simulink library "lic"  (R2021b)
settings: Solver=VariableStepAuto  StartTime=0.0  StopTime=10.0  RelTol=1e-3
undefined symbols (not defined in the file): C_TICK_TIME_S, ENUM_LANEQUALITY_HIGH, ENUM_LANEQUALITY_MEDIUM, ENUM_LFCSTATE_DEGRADED, FALSE, KAPP_VehicleWidth_m, KLIC_C0CrossingThr_m, KLIC_C1Max4Act_rad, KLIC_C2Max4Act_rat, KLIC_C2Max4Disable_rat, KLIC_C2Max4DisableThr_s, KLIC_CalDefaultTLC_s, KLIC_CalTLCMax_s, KLIC_CalTLCMin_s, KLIC_DefaultLaneWidth_m, KLIC_Lane4ActThr_s, KLIC_LaneWidHoldOnTime_s, KLIC_LaneWidRampFinErrThres_m, KLIC_LaneWidRampFinTimeThres_s, KLIC_LaneWidRampInFalRt_mps, KLIC_LaneWidRampInRisRt_mps, KLIC_LaneWidRampOutFalRt_mps, KLIC_LaneWidRampOutRisRt_mps, KLIC_LaneWidthLowThr_m, KLIC_LaneWidthUpThr_m, KLIC_TLCTriggerThrHysis_s, KPER_DefaultLaneWidth_m, MIFO_TLCThr4LKA_s, TRUE
libraries: hcu_lib x33, simulink x8
(part 1 of 2)
settings Model: Creator=power  LastModifiedBy=power

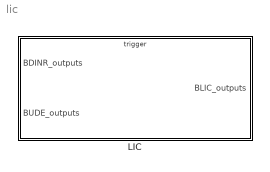
== system lic ==
  LIC : Subsystem

== system lic/LIC ==
  BDINR_outputs : Inport  OutDataTypeStr=Bus: BDINR_outputs
  BUDE_outputs : Inport  Port=2  OutDataTypeStr=Bus: BUDE_outputs
  trig_LIC : TriggerPort  TriggerType=function-call  VariantControl=(inherit)
      settings: AttributesFormatString=State = %<StatesWhenEnabling>
  Bus Creator : BusCreator  Inputs=37  OutDataTypeStr=Bus: BPER_outputs
  Bus Selector1 : BusSelector  OutputSignals=VDINR_CamInternalError_flg,VDINR_LaneQualityL_enum,VDINR_LaneQualityR_enum,VDINR_LaneC0L_m,VDINR_LaneC0R_m,VDINR_LaneC1L_rad,VDINR_LaneC1R_rad,VDINR_LaneC2L_rat,VDINR_LaneC2R_rat,VDINR_LaneC3L_rat,VDINR_LaneC3R_rat,VDINR_TLCL_s,VDINR_TLCLValid_flg,VDINR_TLCR_s,VDINR_TLCRValid_flg,VDINR_VehSpd_mps,VDINR_YawRate_radps,VDINR_ViewRangeEndL_m,VDINR_ViewRangeEndR_m
  Bus Selector2 : BusSelector  OutputSignals=VUDE_NOFTRACKS_num,VUDE_TRACKSX_m,VUDE_TRACKSY_m,VUDE_TRACKSOBST_enum,VUDE_TRACKSVEL_mps,VUDE_TRACKSWIDTH_m,VUDE_TRACKSID_enum,VUDE_TRACKSATT_rad,VUDE_TRACKSEXSPROB_num,VUDE_TRACKSACCEL_mps2,VUDE_RadObjectValid_flg,VUDE_TRACKSRADDYNSTAT_enum,VUDE_CamObstacleValid_flg,VUDE_TRACKSMEDYNSTAT_enum
  lic : Subsystem  TreatAsAtomicUnit=on
  BLIC_outputs : Outport  OutDataTypeStr=Bus: BPER_outputs
  wires:
  Bus Creator/1 -> BLIC_outputs/1  "BLIC_outputs"
  BUDE_outputs/1 -> Bus Selector2/1
  BDINR_outputs/1 -> Bus Selector1/1

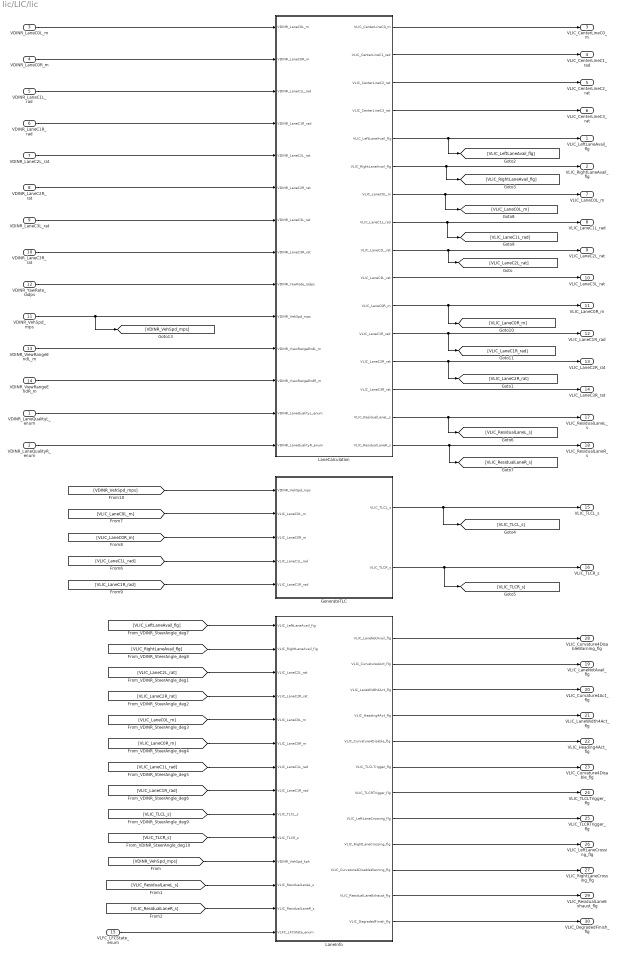
== system lic/LIC/lic ==
  VDINR_LaneQualityL_enum : Inport
  VDINR_LaneQualityR_enum : Inport  Port=2
  VDINR_LaneC0L_m : Inport  Port=3
  VDINR_LaneC0R_m : Inport  Port=4
  VDINR_LaneC1L_rad : Inport  Port=5
  VDINR_LaneC1R_rad : Inport  Port=6
  VDINR_LaneC2L_rat : Inport  Port=7
  VDINR_LaneC2R_rat : Inport  Port=8
  VDINR_LaneC3L_rat : Inport  Port=9
  VDINR_LaneC3R_rat : Inport  Port=10
  VDINR_VehSpd_mps : Inport  Port=11
  VDINR_YawRate_radps : Inport  Port=12
  VDINR_ViewRangeEndL_m : Inport  Port=13
  VDINR_ViewRangeEndR_m : Inport  Port=14
  VLFC_LFCState_enum : Inport  Port=15
  GenerateTLC : Subsystem
  LaneCalculation : Subsystem
  LaneInfo : Subsystem  AncestorBlock=ifo/IFO/ifo/LaneInfo  TreatAsAtomicUnit=on
  VLIC_LeftLaneAvail_flg : Outport
  VLIC_RightLaneAvail_flg : Outport  Port=2
  "VLIC_CenterLineC0_m " : Outport  Port=3
  VLIC_CenterLineC1_rad : Outport  Port=4
  VLIC_CenterLineC2_rat : Outport  Port=5
  VLIC_CenterLineC3_rat : Outport  Port=6
  VLIC_LaneC0L_m : Outport  Port=7
  VLIC_LaneC1L_rad : Outport  Port=8
  VLIC_LaneC2L_rat : Outport  Port=9
  VLIC_LaneC3L_rat : Outport  Port=10
  VLIC_LaneC0R_m : Outport  Port=11
  VLIC_LaneC1R_rad : Outport  Port=12
  VLIC_LaneC2R_rat : Outport  Port=13
  VLIC_LaneC3R_rat : Outport  Port=14
  VLIC_TLCL_s : Outport  Port=15
  VLIC_TLCR_s : Outport  Port=16
  VLIC_ResidualLaneL_s : Outport  Port=17
  VLIC_ResidualLaneR_s : Outport  Port=18
  VLIC_LaneNotAvail_flg : Outport  Port=19
  VLIC_Curvature4Act_flg : Outport  Port=20
  VLIC_LaneWidth4Act_flg : Outport  Port=21
  VLIC_Heading4Act_flg : Outport  Port=22
  VLIC_Curvature4Disable_flg : Outport  Port=23
  VLIC_TLCLTrigger_flg : Outport  Port=24
  VLIC_TLCRTrigger_flg : Outport  Port=25
  VLIC_LeftLaneCrossing_flg : Outport  Port=26
  VLIC_RightLaneCrossing_flg : Outport  Port=27
  VLIC_Curvature4DisableWarning_flg : Outport  Port=28
  VLIC_ResidualLaneExhaust_flg : Outport  Port=29
  VLIC_DegradedFinish_flg : Outport  Port=30
  wires:
  [VDINR_VehSpd_mps] -> GenerateTLC/1(VDINR_VehSpd_mps)
  LaneInfo/1(VLIC_LaneNotAvail_flg) -> VLIC_Curvature4DisableWarning_flg/1
  LaneInfo/10(VLIC_Curvature4DisableWarning_flg) -> VLIC_RightLaneCrossing_flg/1
  LaneInfo/9(VLIC_RightLaneCrossing_flg) -> VLIC_LeftLaneCrossing_flg/1
  LaneInfo/8(VLIC_LeftLaneCrossing_flg) -> VLIC_TLCRTrigger_flg/1
  LaneInfo/7(VLIC_TLCRTrigger_flg) -> VLIC_TLCLTrigger_flg/1
  LaneInfo/6(VLIC_TLCLTrigger_flg) -> VLIC_Curvature4Disable_flg/1
  LaneInfo/5(VLIC_Curvature4Disable_flg) -> VLIC_Heading4Act_flg/1
  LaneInfo/4(VLIC_Heading4Act_flg) -> VLIC_LaneWidth4Act_flg/1
  LaneInfo/3(VLIC_LaneWidth4Act_flg) -> VLIC_Curvature4Act_flg/1
  LaneInfo/2(VLIC_Curvature4Act_flg) -> VLIC_LaneNotAvail_flg/1
  [VDINR_VehSpd_mps] -> LaneInfo/11(VDINR_VehSpd_kph)
  [VLIC_TLCR_s] -> LaneInfo/10(VLIC_TLCR_s)
  [VLIC_TLCL_s] -> LaneInfo/9(VLIC_TLCL_s)
  [VLIC_RightLaneAvail_flg] -> LaneInfo/2("VLIC_RightLaneAvail_fig ")
  [VLIC_LeftLaneAvail_flg] -> LaneInfo/1("VLIC_LeftLaneAvail_fig ")
  [VLIC_LaneC1R_rad] -> LaneInfo/8(VLIC_LaneC1R_rad)
  [VLIC_LaneC1L_rad] -> LaneInfo/7(VLIC_LaneC1L_rad)
  [VLIC_LaneC0R_m] -> LaneInfo/6(VLIC_LaneC0R_m)
  [VLIC_LaneC0L_m] -> LaneInfo/5(VLIC_LaneC0L_m)
  [VLIC_LaneC2R_rat] -> LaneInfo/4(VLIC_LaneC2R_rat)
  [VLIC_LaneC2L_rat] -> LaneInfo/3(VLIC_LaneC2L_rat)
  VDINR_LaneC1L_rad/1 -> LaneCalculation/3(VDINR_LaneC1L_rad)
  VDINR_LaneC2L_rat/1 -> LaneCalculation/5(VDINR_LaneC2L_rat)
  VDINR_LaneC2R_rat/1 -> LaneCalculation/6(VDINR_LaneC2R_rat)
  VDINR_LaneC3L_rat/1 -> LaneCalculation/7(VDINR_LaneC3L_rat)
  VDINR_LaneC3R_rat/1 -> LaneCalculation/8(VDINR_LaneC3R_rat)
  VDINR_LaneQualityL_enum/1 -> LaneCalculation/13(VDINR_LaneQualityL_enum)
  LaneCalculation/1("VLIC_CenterLineC0_m ") -> "VLIC_CenterLineC0_m "/1
  LaneCalculation/2(VLIC_CenterLineC1_rad) -> VLIC_CenterLineC1_rad/1
  LaneCalculation/3(VLIC_CenterLineC2_rat) -> VLIC_CenterLineC2_rat/1
  LaneCalculation/4(VLIC_CenterLineC3_rat) -> VLIC_CenterLineC3_rat/1
  GenerateTLC/1(VLIC_TLCL_s) -> [VLIC_TLCL_s], VLIC_TLCL_s/1
  GenerateTLC/2(VLIC_TLCR_s) -> [VLIC_TLCR_s], VLIC_TLCR_s/1
  [VLIC_LaneC1L_rad] -> GenerateTLC/4(VLIC_LaneC1L_rad)
  [VLIC_LaneC0L_m] -> GenerateTLC/2(VLIC_LaneC0L_m)
  [VLIC_LaneC0R_m] -> GenerateTLC/3(VLIC_LaneC0R_m)
  [VLIC_LaneC1R_rad] -> GenerateTLC/5(VLIC_LaneC1R_rad)
  VDINR_YawRate_radps/1 -> LaneCalculation/9(VDINR_YawRate_radps)
  VDINR_VehSpd_mps/1 -> [VDINR_VehSpd_mps], LaneCalculation/10(VDINR_VehSpd_mps)
  VDINR_ViewRangeEndL_m/1 -> LaneCalculation/11(VDINR_ViewRangeEndL_m)
  VDINR_ViewRangeEndR_m/1 -> LaneCalculation/12(VDINR_ViewRangeEndR_m)
  LaneCalculation/5(VLIC_LeftLaneAvail_flg) -> VLIC_LeftLaneAvail_flg/1, [VLIC_LeftLaneAvail_flg]
  LaneCalculation/6(VLIC_RightLaneAvail_flg) -> VLIC_RightLaneAvail_flg/1, [VLIC_RightLaneAvail_flg]
  VDINR_LaneC1R_rad/1 -> LaneCalculation/4(VDINR_LaneC1R_rad)
  LaneCalculation/7(VLIC_LaneC0L_m) -> [VLIC_LaneC0L_m], VLIC_LaneC0L_m/1
  LaneCalculation/8(VLIC_LaneC1L_rad) -> [VLIC_LaneC1L_rad], VLIC_LaneC1L_rad/1
  LaneCalculation/9(VLIC_LaneC2L_rat) -> VLIC_LaneC2L_rat/1, [VLIC_LaneC2L_rat]
  LaneCalculation/10(VLIC_LaneC3L_rat) -> VLIC_LaneC3L_rat/1
  LaneCalculation/11(VLIC_LaneC0R_m) -> [VLIC_LaneC0R_m], VLIC_LaneC0R_m/1
  LaneCalculation/12(VLIC_LaneC1R_rad) -> [VLIC_LaneC1R_rad], VLIC_LaneC1R_rad/1
  LaneCalculation/13(VLIC_LaneC2R_rat) -> VLIC_LaneC2R_rat/1, [VLIC_LaneC2R_rat]
  LaneCalculation/14(VLIC_LaneC3R_rat) -> VLIC_LaneC3R_rat/1
  VDINR_LaneQualityR_enum/1 -> LaneCalculation/14(VDINR_LaneQualityR_enum)
  VDINR_LaneC0L_m/1 -> LaneCalculation/1(VDINR_LaneC0L_m)
  VDINR_LaneC0R_m/1 -> LaneCalculation/2(VDINR_LaneC0R_m)
  LaneCalculation/15(VLIC_ResidualLaneL_s) -> VLIC_ResidualLaneL_s/1, [VLIC_ResidualLaneL_s]
  LaneCalculation/16(VLIC_ResidualLaneR_s) -> VLIC_ResidualLaneR_s/1, [VLIC_ResidualLaneR_s]
  [VLIC_ResidualLaneL_s] -> LaneInfo/12(VLIC_ResidualLaneL_s)
  [VLIC_ResidualLaneR_s] -> LaneInfo/13(VLIC_ResidualLaneR_s)
  VLFC_LFCState_enum/1 -> LaneInfo/14(VLFC_LFCState_enum)
  LaneInfo/11(VLIC_ResidualLaneExhaust_flg) -> VLIC_ResidualLaneExhaust_flg/1
  LaneInfo/12(VLIC_DegradedFinish_flg) -> VLIC_DegradedFinish_flg/1

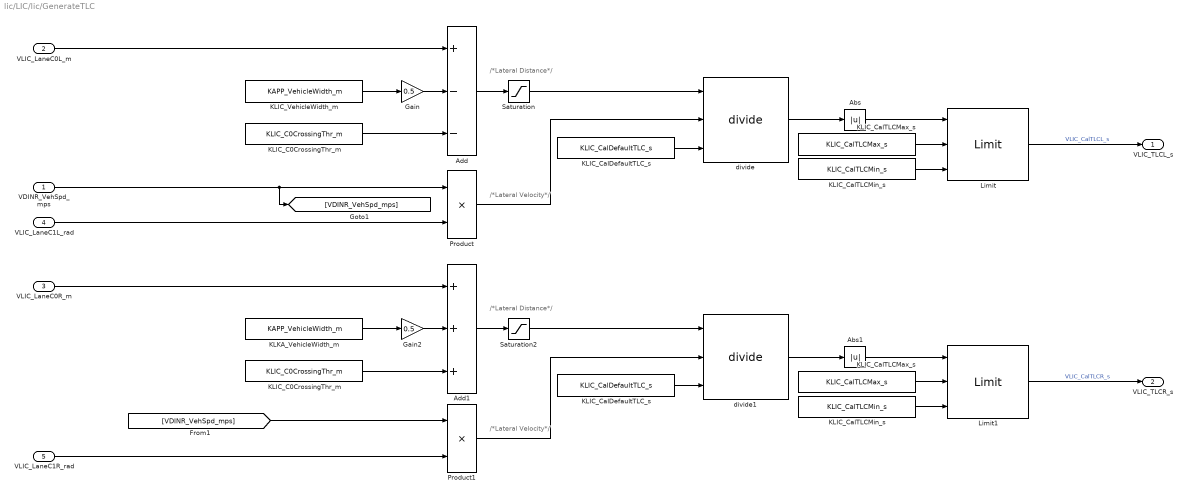
== system lic/LIC/lic/GenerateTLC ==
  note: /*Lateral Velocity*/
  note: /*Lateral Distance*/
  note: /*Lateral Distance*/
  note: /*Lateral Velocity*/
  VDINR_VehSpd_mps : Inport
  VLIC_LaneC0L_m : Inport  Port=2
  VLIC_LaneC0R_m : Inport  Port=3
  VLIC_LaneC1L_rad : Inport  Port=4
  VLIC_LaneC1R_rad : Inport  Port=5
  Abs : Abs
  Abs1 : Abs
  Add : Sum  Inputs=+--
  Add1 : Sum  Inputs=+++
  Gain : Gain  Gain=0.5
  Gain2 : Gain  Gain=0.5
  KLIC_C0CrossingThr_m : Constant  Value=KLIC_C0CrossingThr_m
  "KLIC_C0CrossingThr_m " : Constant  Value=KLIC_C0CrossingThr_m
  KLIC_CalDefaultTLC_s : Constant  Value=KLIC_CalDefaultTLC_s
  "KLIC_CalDefaultTLC_s " : Constant  Value=KLIC_CalDefaultTLC_s
  KLIC_CalTLCMax_s : Constant  Value=KLIC_CalTLCMax_s
  "KLIC_CalTLCMax_s " : Constant  Value=KLIC_CalTLCMax_s
  KLIC_CalTLCMin_s : Constant  Value=KLIC_CalTLCMin_s
  "KLIC_CalTLCMin_s " : Constant  Value=KLIC_CalTLCMin_s
  KLIC_VehicleWidth_m : Constant  Value=KAPP_VehicleWidth_m
  "KLKA_VehicleWidth_m " : Constant  Value=KAPP_VehicleWidth_m
  Limit : hcu_lib/Limit  SystemSampleTime=-1  VariantActivationTime=update diagram  Latency=0  AutoFrameSizeCalculation=off
  Limit1 : hcu_lib/Limit  SystemSampleTime=-1  VariantActivationTime=update diagram  Latency=0  AutoFrameSizeCalculation=off
  Product : Product
  Product1 : Product
  Saturation : Saturate  UpperLimit=inf  LowerLimit=0
  Saturation2 : Saturate  UpperLimit=0  LowerLimit=-inf
  divide : hcu_lib/divide
  divide1 : hcu_lib/divide
  VLIC_TLCL_s : Outport
  VLIC_TLCR_s : Outport  Port=2
  wires:
  Gain/1 -> Add/2
  VLIC_LaneC0L_m/1 -> Add/1
  KLIC_VehicleWidth_m/1 -> Gain/1
  KLIC_C0CrossingThr_m/1 -> Add/3
  VDINR_VehSpd_mps/1 -> Product/1, [VDINR_VehSpd_mps]
  Product/1 -> divide/2
  Add/1 -> Saturation/1
  KLIC_CalDefaultTLC_s/1 -> divide/3
  Saturation/1 -> divide/1
  VLIC_LaneC1L_rad/1 -> Product/2
  divide/1 -> Abs/1
  KLIC_CalTLCMax_s/1 -> Limit/2
  KLIC_CalTLCMin_s/1 -> Limit/3
  Limit/1 -> VLIC_TLCL_s/1  "VLIC_CalTLCL_s"
  Saturation2/1 -> divide1/1
  "KLIC_CalDefaultTLC_s "/1 -> divide1/3
  Add1/1 -> Saturation2/1
  Product1/1 -> divide1/2
  [VDINR_VehSpd_mps] -> Product1/1
  "KLIC_C0CrossingThr_m "/1 -> Add1/3
  "KLKA_VehicleWidth_m "/1 -> Gain2/1
  Gain2/1 -> Add1/2
  VLIC_LaneC0R_m/1 -> Add1/1
  "KLIC_CalTLCMax_s "/1 -> Limit1/2
  "KLIC_CalTLCMin_s "/1 -> Limit1/3
  Limit1/1 -> VLIC_TLCR_s/1  "VLIC_CalTLCR_s"
  divide1/1 -> Abs1/1
  VLIC_LaneC1R_rad/1 -> Product1/2
  Abs/1 -> Limit/1
  Abs1/1 -> Limit1/1

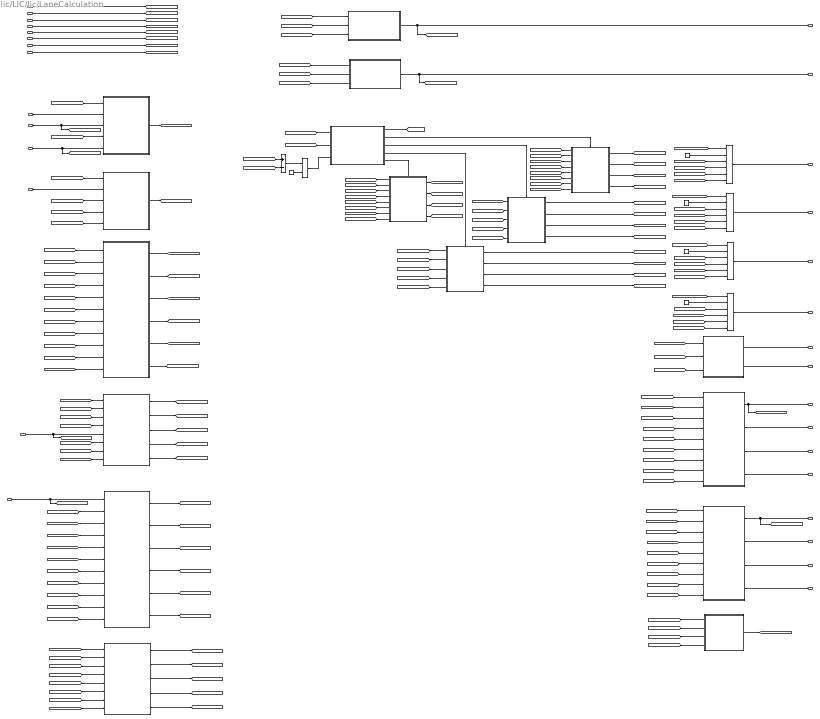
== system lic/LIC/lic/LaneCalculation ==
  VDINR_LaneC0L_m : Inport
  VDINR_LaneC0R_m : Inport  Port=2
  VDINR_LaneC1L_rad : Inport  Port=3
  VDINR_LaneC1R_rad : Inport  Port=4
  VDINR_LaneC2L_rat : Inport  Port=5
  VDINR_LaneC2R_rat : Inport  Port=6
  VDINR_LaneC3L_rat : Inport  Port=7
  VDINR_LaneC3R_rat : Inport  Port=8
  VDINR_YawRate_radps : Inport  Port=9
  VDINR_VehSpd_mps : Inport  Port=10
  VDINR_ViewRangeEndL_m : Inport  Port=11
  VDINR_ViewRangeEndR_m : Inport  Port=12
  VDINR_LaneQualityL_enum : Inport  Port=13
  VDINR_LaneQualityR_enum : Inport  Port=14
  Add2 : Sum  Inputs=+-
  C1L_Bias : Subsystem  AncestorBlock=per/PER/per/Lane_Process/C1L_Bias  TreatAsAtomicUnit=on
  C1R_Bias : Subsystem  AncestorBlock=per/PER/per/Lane_Process/C1R_Bias  TreatAsAtomicUnit=on
  C2diff_thr : Constant  Value=0.01
  Constant{,1..3} (4 alike) : Constant  Value=0  OutDataTypeStr=single
  GenerateLeftLane : Subsystem
  GenerateRightLane : Subsystem
  LR_Available : Subsystem  TreatAsAtomicUnit=on
  LR_NotAvailable : Subsystem  TreatAsAtomicUnit=on
  LaneL_estimator : Subsystem  TreatAsAtomicUnit=on
  LaneR_estimator : Subsystem  TreatAsAtomicUnit=on
  LaneResidual_Calculation : Subsystem
  LaneWidth : Subsystem
  Lane_status : Stateflow chart  TreatAsAtomicUnit=on
  Multiport Switch{,1..3} (4 alike) : MultiPortSwitch  DataPortOrder=Zero-based contiguous  Inputs=5  zeroidx=on
  OnlyL_Available : Subsystem  TreatAsAtomicUnit=on
  OnlyR_Available : Subsystem  TreatAsAtomicUnit=on
  Relational Operator : RelationalOperator  Operator=<=  OutDataTypeStr=boolean  RndMeth=Nearest
  UsingRawLaneL : Subsystem
  UsingRawLaneR : Subsystem
  Using_estimator_LeftLane : Subsystem
  Using_estimator_RightLane : Subsystem
  "VLIC_CenterLineC0_m " : Outport
  VLIC_CenterLineC1_rad : Outport  Port=2
  VLIC_CenterLineC2_rat : Outport  Port=3
  VLIC_CenterLineC3_rat : Outport  Port=4
  VLIC_LeftLaneAvail_flg : Outport  Port=5
  VLIC_RightLaneAvail_flg : Outport  Port=6
  VLIC_LaneC0L_m : Outport  Port=7
  VLIC_LaneC1L_rad : Outport  Port=8
  VLIC_LaneC2L_rat : Outport  Port=9
  VLIC_LaneC3L_rat : Outport  Port=10
  VLIC_LaneC0R_m : Outport  Port=11
  VLIC_LaneC1R_rad : Outport  Port=12
  VLIC_LaneC2R_rat : Outport  Port=13
  VLIC_LaneC3R_rat : Outport  Port=14
  VLIC_ResidualLaneL_s : Outport  Port=15
  VLIC_ResidualLaneR_s : Outport  Port=16
  wires:
  [VDINR_VehSpd_mps] -> LaneL_estimator/6(VDINR_VehSpd_mps)
  C1R_Bias/1(VLIC_LaneC1RUpdate_rad) -> [VLIC_LaneC1RUpdate_rad]
  C1L_Bias/1(VLIC_LaneC1LUpdate_rad) -> [VLIC_LaneC1LUpdate_rad]
  [VDINR_LaneC2R_rat] -> C1R_Bias/4(VDINR_LaneC2R_rat)
  [VDINR_VehSpd_mps] -> C1R_Bias/3(VDINR_VehSpd_mps)
  [VDINR_LaneC0R_m] -> C1R_Bias/1(VDINR_LaneC0R_m)
  [VDINR_LaneQualityR_enum] -> C1R_Bias/5(VDINR_LaneQualityL_enum)
  [VDINR_LaneQualityL_enum] -> UsingRawLaneL/1(VDINR_LaneQualityL_enum)
  [VDINR_LaneC2L_rat] -> C1L_Bias/4(VDINR_LaneC2L_rat)
  VDINR_VehSpd_mps/1 -> C1L_Bias/3(VDINR_VehSpd_mps), [VDINR_VehSpd_mps]
  [VDINR_LaneC0L_m] -> C1L_Bias/1(VDINR_LaneC0L_m)
  [VDINR_LaneC0R_m] -> LR_Available/2(VDINR_LaneC0R_m)
  [VDINR_LaneC0L_m] -> LR_Available/1(VDINR_LaneC0L_m)
  [VDINR_LaneC2L_rat] -> OnlyL_Available/4(VDINR_LaneC2L_rat)
  OnlyL_Available/1(VLIC_LCenterLineC0_m) -> [VLIC_LCenterLineC0_m]
  [VDINR_LaneC3L_rat] -> OnlyL_Available/5(VDINR_LaneC3L_rat)
  LR_Available/1(VLIC_RLCenterLineC0_m) -> [VLIC_RLCenterLineC0_m]
  OnlyR_Available/1(VLIC_RCenterLineC0_m) -> [VLIC_RCenterLineC0_m]
  LR_Available/2(VLIC_RLCenterLineC1_rad) -> [VLIC_RLCenterLineC1_rad]
  OnlyR_Available/2(VLIC_RCenterLineC1_rad) -> [VLIC_RCenterLineC1_rad]
  [VLIC_LaneWidth_m] -> OnlyL_Available/1(VLIC_LaneWidth_m)
  OnlyR_Available/3(VLIC_RCenterLineC2_rat) -> [VLIC_RCenterLineC2_rat]
  OnlyR_Available/4(VLIC_RCenterLineC3_rat) -> [VLIC_RCenterLineC3_rat]
  [VLIC_LaneWidth_m] -> OnlyR_Available/1(VLIC_LaneWidth_m)
  LR_Available/3(VLIC_RLCenterLineC2_rat) -> [VLIC_RLCenterLineC2_rat]
  LR_Available/4(VLIC_RLCenterLineC3_rat) -> [VLIC_RLCenterLineC3_rat]
  [VDINR_LaneC0R_m] -> OnlyR_Available/2(VDINR_LaneC0R_m)
  [VDINR_LaneC0L_m] -> OnlyL_Available/2(VDINR_LaneC0L_m)
  [VLIC_LaneC1RUpdate_rad] -> OnlyR_Available/3(VDINR_LaneC1R_rad)
  [VDINR_LaneC2R_rat] -> OnlyR_Available/4(VDINR_LaneC2R_rat)
  [VDINR_LaneC3R_rat] -> OnlyR_Available/5(VDINR_LaneC3R_rat)
  OnlyL_Available/4(VLIC_LCenterLineC3_rat) -> [VLIC_LCenterLineC3_rat]
  OnlyL_Available/3(VLIC_LCenterLineC2_rat) -> [VLIC_LCenterLineC2_rat]
  OnlyL_Available/2(VLIC_LCenterLineC1_rad) -> [VLIC_LCenterLineC1_rad]
  [VLIC_LaneC1LUpdate_rad] -> OnlyL_Available/3(VDINR_LaneC1L_rad)
  [VDINR_LaneC3R_rat] -> LR_Available/8(VDINR_LaneC3R_rat)
  [VDINR_LaneC3L_rat] -> LR_Available/7(VDINR_LaneC3L_rat)
  [VDINR_LaneC2L_rat] -> LR_Available/5(VDINR_LaneC2L_rat)
  [VLIC_LaneC1RUpdate_rad] -> LR_Available/4(VDINR_LaneC1R_rad)
  [VLIC_LaneC1LUpdate_rad] -> LR_Available/3(VDINR_LaneC1L_rad)
  [VDINR_LaneC2R_rat] -> LR_Available/6(VDINR_LaneC2R_rat)
  VDINR_LaneC0L_m/1 -> [VDINR_LaneC0L_m]
  VDINR_LaneC0R_m/1 -> [VDINR_LaneC0R_m]
  VDINR_LaneC2L_rat/1 -> [VDINR_LaneC2L_rat]
  VDINR_LaneC2R_rat/1 -> [VDINR_LaneC2R_rat]
  VDINR_LaneC3L_rat/1 -> [VDINR_LaneC3L_rat]
  VDINR_LaneC3R_rat/1 -> [VDINR_LaneC3R_rat]
  Lane_status/1(SWCase) -> [SWCase]  "SW_CASE"
  Lane_status/2(LR_avail) -> LR_Available/Enable
  Lane_status/4(L_avail) -> OnlyL_Available/Enable
  Lane_status/3(R_avail) -> OnlyR_Available/Enable
  [SWCase] -> Multiport Switch/1
  [VLIC_RLCenterLineC0_m] -> Multiport Switch/3
  [VLIC_RCenterLineC0_m] -> Multiport Switch/4
  [VLIC_LCenterLineC0_m] -> Multiport Switch/5
  Constant/1 -> Multiport Switch/2
  [SWCase] -> Multiport Switch1/1
  [VLIC_RLCenterLineC1_rad] -> Multiport Switch1/3
  [VLIC_RCenterLineC1_rad] -> Multiport Switch1/4
  [VLIC_LCenterLineC1_rad] -> Multiport Switch1/5
  Constant1/1 -> Multiport Switch1/2
  [SWCase] -> Multiport Switch2/1
  Constant2/1 -> Multiport Switch2/2
  [VLIC_RLCenterLineC2_rat] -> Multiport Switch2/3
  [VLIC_RCenterLineC2_rat] -> Multiport Switch2/4
  [SWCase] -> Multiport Switch3/1
  Constant3/1 -> Multiport Switch3/2
  [VLIC_RLCenterLineC3_rat] -> Multiport Switch3/3
  [VLIC_RCenterLineC3_rat] -> Multiport Switch3/4
  [OptLaneC0L] -> LaneL_estimator/1(OptLaneC0L)
  [OptLaneC1L] -> LaneL_estimator/2(OptLaneC1L)
  [OptLaneC2L] -> LaneL_estimator/3(OptLaneC2L)
  [OptLaneC3L] -> LaneL_estimator/4(OptLaneC3L)
  VDINR_ViewRangeEndL_m/1 -> [VDINR_ViewRangeEndL_m]
  VDINR_ViewRangeEndR_m/1 -> [VDINR_ViewRangeEndR_m]
  [OptLaneC0R] -> LaneR_estimator/1(OptLaneC0R)
  [OptLaneC1R] -> LaneR_estimator/2(OptLaneC1R)
  [OptLaneC2R] -> LaneR_estimator/3(OptLaneC2R)
  [OptLaneC3R] -> LaneR_estimator/4(OptLaneC3R)
  [VDINR_YawRate_radps] -> LaneR_estimator/5(VDINR_YawRate_radps)
  [VDINR_VehSpd_mps] -> LaneR_estimator/6(VDINR_VehSpd_mps)
  Multiport Switch/1 -> "VLIC_CenterLineC0_m "/1  "VLIC_CenterLineC0_m"
  Multiport Switch1/1 -> VLIC_CenterLineC1_rad/1  "VLIC_CenterLineC1_rad"
  Multiport Switch2/1 -> VLIC_CenterLineC2_rat/1  "VLIC_CenterLineC2_rat"
  Multiport Switch3/1 -> VLIC_CenterLineC3_rat/1  "VLIC_CenterLineC3_rat"
  [VLIC_LeftLaneAvail_flg] -> Lane_status/1(VLIC_LeftLaneAvail_fig)
  [VLIC_RightLaneAvail_flg] -> Lane_status/2(VLIC_RightLaneAvail_fig)
  Lane_status/5(NO_avail) -> LR_NotAvailable/Enable
  [VLIC_EstLaneC0L_m] -> LR_NotAvailable/1(VLIC_EstLaneC0L_m)
  [VLIC_EstLaneC0R_m] -> LR_NotAvailable/2(VLIC_EstLaneC0R_m)
  [VLIC_EstLaneC1L_rad] -> LR_NotAvailable/3(VLIC_EstLaneC1L_rad)
  [VLIC_EstLaneC1R_rad] -> LR_NotAvailable/4(VLIC_EstLaneC1R_rad)
  [VLIC_EstLaneC2R_rat] -> LR_NotAvailable/6(VLIC_EstLaneC2R_rat)
  [VLIC_EstLaneC3R_rat] -> LR_NotAvailable/8(VLIC_EstLaneC3R_rat)
  [VLIC_EstLaneC3L_rat] -> LR_NotAvailable/7(VLIC_EstLaneC3L_rat)
  [VLIC_EstLaneC2L_rat] -> LR_NotAvailable/5(VLIC_EstLaneC2L_rat)
  LR_NotAvailable/1(VLIC_EstCenterLineC0_m) -> [VLIC_EstCenterLineC0_m]
  LR_NotAvailable/2(VLIC_EstCenterLineC1_rad) -> [VLIC_EstCenterLineC1_rad]
  LR_NotAvailable/3(VLIC_EstCenterLineC2_rat) -> [VLIC_EstCenterLineC2_rat]
  LR_NotAvailable/4(VLIC_EstCenterLineC3_rat) -> [VLIC_EstCenterLineC3_rat]
  [VLIC_EstCenterLineC0_m] -> Multiport Switch/6
  LaneL_estimator/5(VLIC_EstViewRangeEndL_m) -> [VLIC_EstViewRangeEndL_m]
  LaneL_estimator/4(VLIC_EstLaneC3L_rat) -> [VLIC_EstLaneC3L_rat]
  LaneL_estimator/3(VLIC_EstLaneC2L_rat) -> [VLIC_EstLaneC2L_rat]
  LaneL_estimator/2(VLIC_EstLaneC1L_rad) -> [VLIC_EstLaneC1L_rad]
  LaneL_estimator/1(VLIC_EstLaneC0L_m) -> [VLIC_EstLaneC0L_m]
  [VLIC_EstCenterLineC1_rad] -> Multiport Switch1/6
  [VLIC_EstCenterLineC2_rat] -> Multiport Switch2/6
  [VLIC_LCenterLineC2_rat] -> Multiport Switch2/5
  [VLIC_EstCenterLineC3_rat] -> Multiport Switch3/6
  [VLIC_LCenterLineC3_rat] -> Multiport Switch3/5
  [OptViewRange_L] -> LaneL_estimator/7(OptViewRange_L)
  [OptViewRange_R] -> LaneR_estimator/7(OptViewRange_R)
  [UsingRawLaneL_flg] -> LaneL_estimator/8(UsingRawLaneL_flg)
  [UsingRawLaneR_flg] -> LaneR_estimator/8(UsingRawLaneR_flg)
  VDINR_YawRate_radps/1 -> LaneL_estimator/5(VDINR_YawRate_radps), [VDINR_YawRate_radps]
  Using_estimator_LeftLane/1(VLIC_LeftLaneAvail_flg) -> VLIC_LeftLaneAvail_flg/1, [VLIC_LeftLaneAvail_flg]
  [VDINR_LaneQualityL_enum] -> Using_estimator_LeftLane/1(VDINR_LaneQualityL_enum)
  [VDINR_ViewRangeEndL_m] -> Using_estimator_LeftLane/2(VDINR_ViewRangeEndL_m)
  [VLIC_EstViewRangeEndL_m] -> Using_estimator_LeftLane/3(VLIC_EstViewRangeEndL_m)
  VDINR_LaneQualityL_enum/1 -> C1L_Bias/5(VDINR_LaneQualityL_enum), [VDINR_LaneQualityL_enum]
  [VDINR_ViewRangeEndL_m] -> UsingRawLaneL/2(VDINR_ViewRangeEndL_m)
  [VLIC_EstViewRangeEndL_m] -> UsingRawLaneL/3(VLIC_EstViewRangeEndL_m)
  VDINR_LaneQualityR_enum/1 -> UsingRawLaneR/1(VDINR_LaneQualityR_enum), [VDINR_LaneQualityR_enum]
  Using_estimator_RightLane/1(VLIC_RightLaneAvail_flg) -> [VLIC_RightLaneAvail_flg], VLIC_RightLaneAvail_flg/1
  [VDINR_LaneQualityR_enum] -> Using_estimator_RightLane/1(VDINR_LaneQualityR_enum)
  [VDINR_ViewRangeEndR_m] -> Using_estimator_RightLane/2(VDINR_ViewRangeEndR_m)
  [VLIC_EstViewRangeEndR_m] -> Using_estimator_RightLane/3(VLIC_EstViewRangeEndR_m)
  [VDINR_LaneC0L_m] -> GenerateLeftLane/1(VDINR_LaneC0L_m)
  [VLIC_EstLaneC0L_m] -> GenerateLeftLane/2(VLIC_EstLaneC0L_m)
  [VLIC_LaneC1LUpdate_rad] -> GenerateLeftLane/3(VDINR_LaneC1L_rad)
  [VLIC_EstLaneC1L_rad] -> GenerateLeftLane/4(VLIC_EstLaneC1L_rad)
  [VDINR_LaneC2L_rat] -> GenerateLeftLane/5(VDINR_LaneC2L_rat)
  [VLIC_EstLaneC2L_rat] -> GenerateLeftLane/6(VLIC_EstLaneC2L_rat)
  [VDINR_LaneC3L_rat] -> GenerateLeftLane/7(VDINR_LaneC3L_rat)
  [VLIC_EstLaneC3L_rat] -> GenerateLeftLane/8(VLIC_EstLaneC3L_rat)
  GenerateLeftLane/1(VLIC_LaneC0L_m) -> [VLIC_LaneC0L_m], VLIC_LaneC0L_m/1
  GenerateLeftLane/2(VLIC_LaneC1L_rad) -> VLIC_LaneC1L_rad/1
  GenerateLeftLane/3(VLIC_LaneC2L_rat) -> VLIC_LaneC2L_rat/1
  GenerateLeftLane/4(VLIC_LaneC3L_rat) -> VLIC_LaneC3L_rat/1
  GenerateRightLane/1(VLIC_LaneC0R_m) -> [VLIC_LaneC0R_m], VLIC_LaneC0R_m/1
  GenerateRightLane/2(VLIC_LaneC1R_rad) -> VLIC_LaneC1R_rad/1
  GenerateRightLane/3(VLIC_LaneC2R_rat) -> VLIC_LaneC2R_rat/1
  GenerateRightLane/4(VLIC_LaneC3R_rat) -> VLIC_LaneC3R_rat/1
  [VLIC_EstLaneC1R_rad] -> GenerateRightLane/4(VLIC_EstLaneC1R_rad)
  [VDINR_LaneC2R_rat] -> GenerateRightLane/5(VDINR_LaneC2R_rat)
  [VLIC_RightLaneAvail_flg] -> GenerateRightLane/9(VLIC_RightLaneAvail_flg)
  [VLIC_EstLaneC3L_rat] -> GenerateRightLane/8(VLIC_EstLaneC3R_rat)
  [VLIC_EstLaneC2R_rat] -> GenerateRightLane/6(VLIC_EstLaneC2R_rat)
  [VDINR_LaneC3R_rat] -> GenerateRightLane/7(VDINR_LaneC3R_rat)
  [VLIC_EstLaneC0R_m] -> GenerateRightLane/2(VLIC_EstLaneC0R_m)
  [VLIC_LaneC1RUpdate_rad] -> GenerateRightLane/3(VDINR_LaneC1R_rad)
  [VDINR_LaneC0R_m] -> GenerateRightLane/1(VDINR_LaneC0R_m)
  [VLIC_EstLaneC0L_m] -> UsingRawLaneL/5(VLIC_EstLaneC0L_m)
  [VDINR_LaneC0L_m] -> UsingRawLaneL/4(VDINR_LaneC0L_m)
  [VLIC_EstLaneC1L_rad] -> UsingRawLaneL/7(VLIC_EstLaneC1L_rad)
  [VLIC_LaneC1LUpdate_rad] -> UsingRawLaneL/6(VDINR_LaneC1L_rad)
  [VLIC_EstLaneC2L_rat] -> UsingRawLaneL/9(VLIC_EstLaneC2L_rat)
  [VDINR_LaneC2L_rat] -> UsingRawLaneL/8(VDINR_LaneC2L_rat)
  [VLIC_EstLaneC3L_rat] -> UsingRawLaneL/11(VLIC_EstLaneC3L_rat)
  [VDINR_LaneC3L_rat] -> UsingRawLaneL/10(VDINR_LaneC3L_rat)
  UsingRawLaneL/2(OptLaneC0L) -> [OptLaneC0L]
  UsingRawLaneL/3(OptLaneC1L) -> [OptLaneC1L]
  UsingRawLaneL/4(OptLaneC2L) -> [OptLaneC2L]
  UsingRawLaneL/5(OptLaneC3L) -> [OptLaneC3L]
  UsingRawLaneL/6(OptViewRange_L) -> [OptViewRange_L]
  UsingRawLaneL/1(UsingRawLaneL_flg) -> [UsingRawLaneL_flg]
  [VDINR_ViewRangeEndR_m] -> UsingRawLaneR/2(VDINR_ViewRangeEndR_m)
  [VLIC_EstViewRangeEndR_m] -> UsingRawLaneR/3(VLIC_EstViewRangeEndR_m)
  UsingRawLaneR/1(UsingRawLaneR_flg) -> [UsingRawLaneR_flg]
  [VLIC_EstLaneC0R_m] -> UsingRawLaneR/5(VLIC_EstLaneC0R_m)
  [VDINR_LaneC0R_m] -> UsingRawLaneR/4(VDINR_LaneC0R_m)
  [VLIC_EstLaneC1R_rad] -> UsingRawLaneR/7(VLIC_EstLaneC1R_rad)
  [VLIC_LaneC1RUpdate_rad] -> UsingRawLaneR/6(VDINR_LaneC1R_rad)
  [VDINR_LaneC2R_rat] -> UsingRawLaneR/8(VDINR_LaneC2R_rat)
  [VLIC_EstLaneC2R_rat] -> UsingRawLaneR/9(VLIC_EstLaneC2R_rat)
  [VDINR_LaneC3R_rat] -> UsingRawLaneR/10(VDINR_LaneC3R_rat)
  [VLIC_EstLaneC3R_rat] -> UsingRawLaneR/11(VLIC_EstLaneC3R_rat)
  UsingRawLaneR/2(OptLaneC0R) -> [OptLaneC0R]
  UsingRawLaneR/3(OptLaneC1R) -> [OptLaneC1R]
  UsingRawLaneR/4(OptLaneC2R) -> [OptLaneC2R]
  UsingRawLaneR/5(OptLaneC3R) -> [OptLaneC3R]
  LaneR_estimator/1(VLIC_EstLaneC0R_m) -> [VLIC_EstLaneC0R_m]
  LaneR_estimator/2(VLIC_EstLaneC1R_rad) -> [VLIC_EstLaneC1R_rad]
  LaneR_estimator/3(VLIC_EstLaneC2R_rat) -> [VLIC_EstLaneC2R_rat]
  LaneR_estimator/4(VLIC_EstLaneC3R_rat) -> [VLIC_EstLaneC3R_rat]
  LaneR_estimator/5(VLIC_EstViewRangeEndR_m) -> [VLIC_EstViewRangeEndR_m]
  UsingRawLaneR/6(OptViewRange_R) -> [OptViewRange_R]
  [VLIC_LeftLaneAvail_flg] -> LaneWidth/1(VLIC_LeftLaneAvail_flg)
  [VLIC_RightLaneAvail_flg] -> LaneWidth/2(VLIC_RightLaneAvail_flg)
  [VLIC_LaneC0R_m] -> LaneWidth/4(VLIC_LaneC0R_m)
  [VLIC_LaneC0L_m] -> LaneWidth/3(VLIC_LaneC0L_m)
  LaneWidth/1(VLIC_LaneWidth_m) -> [VLIC_LaneWidth_m]
  VDINR_LaneC1L_rad/1 -> C1L_Bias/2(VDINR_LaneC1L_rad)
  VDINR_LaneC1R_rad/1 -> C1R_Bias/2(VDINR_LaneC1R_rad)
  [VLIC_EstViewRangeEndL_m] -> LaneResidual_Calculation/1(VLIC_EstViewRangeEndL_m)
  [VDINR_VehSpd_mps] -> LaneResidual_Calculation/2(VDINR_VehSpd_mps)
  [VLIC_EstViewRangeEndR_m] -> LaneResidual_Calculation/3(VLIC_EstViewRangeEndR_m)
  LaneResidual_Calculation/1(VLIC_ResidualLaneL_s) -> VLIC_ResidualLaneL_s/1
  LaneResidual_Calculation/2(VLIC_ResidualLaneR_s) -> VLIC_ResidualLaneR_s/1
  [VDINR_LaneC2L_rat] -> Add2/1
  [VDINR_LaneC2R_rat] -> Add2/2
  Add2/1 -> Relational Operator/1
  C2diff_thr/1 -> Relational Operator/2
  Relational Operator/1 -> Lane_status/3(VLIC_C2Diff_flg)
  [VLIC_LeftLaneAvail_flg] -> GenerateLeftLane/9(VLIC_LeftLaneAvail_flg)

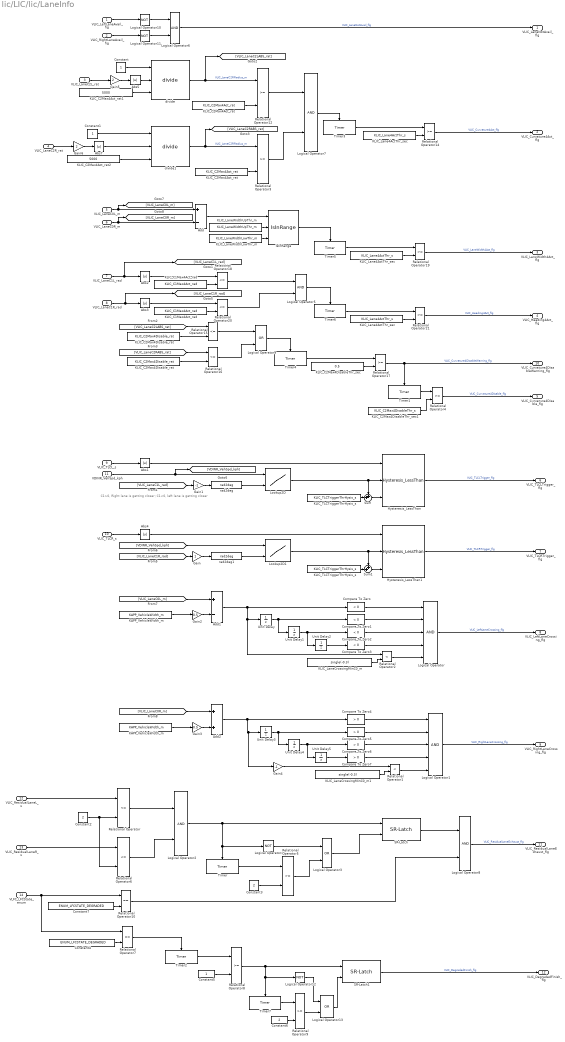
== system lic/LIC/lic/LaneInfo ==
  note: C1>0, Right lane is getting closer; C1<0, left lane is getting closer
  "VLIC_LeftLaneAvail_fig " : Inport
  "VLIC_RightLaneAvail_fig " : Inport  Port=2
  VLIC_LaneC2L_rat : Inport  Port=3
  VLIC_LaneC2R_rat : Inport  Port=4
  VLIC_LaneC0L_m : Inport  Port=5
  VLIC_LaneC0R_m : Inport  Port=6
  VLIC_LaneC1L_rad : Inport  Port=7
  VLIC_LaneC1R_rad : Inport  Port=8
  VLIC_TLCL_s : Inport  Port=9
  VLIC_TLCR_s : Inport  Port=10
  VDINR_VehSpd_kph : Inport  Port=11
  VLIC_ResidualLaneL_s : Inport  Port=12
  VLIC_ResidualLaneR_s : Inport  Port=13
  VLFC_LFCState_enum : Inport  Port=14
  Abs{1..5,7} (6 alike) : Abs
  Add : Sum  Inputs=+-
  Add1 : Sum  Inputs=+-
  Add2 : Sum
  Compare To Zero{,1..3} (4 alike) : simulink/Logic and Bit Operations/Compare To Zero  relop=<  OutDataTypeStr=boolean
  Compare To Zero{4..7} (4 alike) : simulink/Logic and Bit Operations/Compare To Zero  relop=>  OutDataTypeStr=boolean
  Constant : Constant  OutDataTypeStr=single
  Constant1 : Constant  OutDataTypeStr=single
  Constant2 : Constant  Value=2  OutDataTypeStr=single
  Constant3 : Constant  Value=2  OutDataTypeStr=single
  Constant4 : Constant  Value=ENUM_LFCSTATE_DEGRADED
  Constant5 : Constant  OutDataTypeStr=single
  Constant6 : Constant  Value=2  OutDataTypeStr=single
  Constant7 : Constant  Value=ENUM_LFCSTATE_DEGRADED
  Gain : Gain
  Gain1 : Gain  Gain=-1
  Gain2 : Gain  Gain=0.5
  Gain3 : Gain  Gain=0.5
  Gain4 : Gain  Gain=-1
  Gain5 : Gain  Gain=2
  Gain6 : Gain  Gain=2
  Hysteresis_LessThan : hcu_lib/Hysteresis_LessThan  SystemSampleTime=-1  VariantActivationTime=update diagram  Latency=0  AutoFrameSizeCalculation=off
  Hysteresis_LessThan1 : hcu_lib/Hysteresis_LessThan  SystemSampleTime=-1  VariantActivationTime=update diagram  Latency=0  AutoFrameSizeCalculation=off
  IsInRange : hcu_lib/IsInRange  SystemSampleTime=-1  VariantActivationTime=update diagram  Latency=0  AutoFrameSizeCalculation=off
  KAPP_VehicleWidth_m : Constant  Value=KAPP_VehicleWidth_m
  "KAPP_VehicleWidth_m " : Constant  Value=KAPP_VehicleWidth_m
  KLIC_C1Max4Act_rad : Constant  Value=KLIC_C1Max4Act_rad
  "KLIC_C1Max4Act_rad " : Constant  Value=KLIC_C1Max4Act_rad
  KLIC_C2Max4Act_rat : Constant  Value=KLIC_C2Max4Act_rat
  "KLIC_C2Max4Act_rat " : Constant  Value=KLIC_C2Max4Act_rat
  KLIC_C2Max4Act_rat1 : Constant  Value=5000  OutDataTypeStr=single
  KLIC_C2Max4Act_rat2 : Constant  Value=5000  OutDataTypeStr=single
  KLIC_C2Max4DisableThr_sec : Constant  Value=0.5
  KLIC_C2Max4DisableThr_sec1 : Constant  Value=KLIC_C2Max4DisableThr_s
  KLIC_C2Max4Disable_rat : Constant  Value=KLIC_C2Max4Disable_rat
  "KLIC_C2Max4Disable_rat " : Constant  Value=KLIC_C2Max4Disable_rat
  KLIC_Lane4ActThr_sec : Constant  Value=KLIC_Lane4ActThr_s
  "KLIC_Lane4ActThr_sec " : Constant  Value=KLIC_Lane4ActThr_s
  "KLIC_Lane4ActThr_sec   " : Constant  Value=KLIC_Lane4ActThr_s
  KLIC_LaneCrossingMinC0_m : Constant  Value=single(-0.3)
  KLIC_LaneCrossingMinC0_m1 : Constant  Value=single(-0.3)
  KLIC_LaneWidthLowThr_m : Constant  Value=KLIC_LaneWidthLowThr_m  OutDataTypeStr=single
  KLIC_LaneWidthUpThr_m : Constant  Value=KLIC_LaneWidthUpThr_m  OutDataTypeStr=single
  KLIC_TLCTriggerThrHysis_s : Constant  Value=KLIC_TLCTriggerThrHysis_s
  "KLIC_TLCTriggerThrHysis_s " : Constant  Value=KLIC_TLCTriggerThrHysis_s
  Logical Operator : Logic  Inputs=5  AllPortsSameDT=off  OutDataTypeStr=boolean
  Logical Operator1 : Logic  Inputs=5  AllPortsSameDT=off  OutDataTypeStr=boolean
  Logical Operator{4,10..12} (4 alike) : Logic  Operator=NOT  AllPortsSameDT=off  OutDataTypeStr=boolean
  Logical Operator13 : Logic  Operator=OR  AllPortsSameDT=off  OutDataTypeStr=boolean
  Logical Operator{2,5..8} (5 alike) : Logic  AllPortsSameDT=off  OutDataTypeStr=boolean
  Logical Operator3 : Logic  Operator=OR  AllPortsSameDT=off  OutDataTypeStr=boolean
  Logical Operator9 : Logic  Operator=OR  AllPortsSameDT=off  OutDataTypeStr=boolean
  Lookup2D : Lookup2D  RowIndex=AIFO_TLCThrVehSpd_X_kph  ColumnIndex=AIFO_TLCThrHeading_Y_deg  Table=MIFO_TLCThr4LKA_s  LookUpMeth=Interpolation-Use End Values  OutDataTypeStr=single
      settings: AttributesFormatString=|
      | <row=%<RowIndex>>
      | <column=%<ColumnIndex>>
      | <table=%<Table>>
  Lookup2D1 : Lookup2D  RowIndex=AIFO_TLCThrVehSpd_X_kph  ColumnIndex=AIFO_TLCThrHeading_Y_deg  Table=MIFO_TLCThr4LKA_s  LookUpMeth=Interpolation-Use End Values  OutDataTypeStr=single
      settings: AttributesFormatString=|
      | <row=%<RowIndex>>
      | <column=%<ColumnIndex>>
      | <table=%<Table>>
  Relational Operator{,6,15..16,18,20} (6 alike) : RelationalOperator  Operator=<=  OutDataTypeStr=boolean  RndMeth=Nearest
  Relational Operator1 : RelationalOperator  Operator=<  OutDataTypeStr=boolean  RndMeth=Nearest
  Relational Operator10 : RelationalOperator  Operator===  OutDataTypeStr=boolean  RndMeth=Nearest
  Relational Operator{3..5,8..9,12,14,17,19,21} (10 alike) : RelationalOperator  OutDataTypeStr=boolean  RndMeth=Nearest
  Relational Operator2 : RelationalOperator  Operator=<  OutDataTypeStr=boolean  RndMeth=Nearest
  Relational Operator7 : RelationalOperator  Operator===  OutDataTypeStr=boolean  RndMeth=Nearest
  SR-Latch : hcu_lib/SR-Latch  SystemSampleTime=-1  VariantActivationTime=update diagram  Latency=0  AutoFrameSizeCalculation=off
  SR-Latch1 : hcu_lib/SR-Latch  SystemSampleTime=-1  VariantActivationTime=update diagram  Latency=0  AutoFrameSizeCalculation=off
  Sum : Sum  Inputs=++|
  Sum1 : Sum  Inputs=++|
  Timer{,1..7} (8 alike) : hcu_lib/Timer  SystemSampleTime=-1  VariantActivationTime=update diagram  Latency=0  AutoFrameSizeCalculation=off
  Unit Delay{,1..5} (6 alike) : UnitDelay  SampleTime=-1  HasFrameUpgradeWarning=on
  divide : hcu_lib/divide
  divide1 : hcu_lib/divide
  rad2deg : hcu_lib/rad2deg
  rad2deg1 : hcu_lib/rad2deg
  VLIC_LaneNotAvail_flg : Outport
  VLIC_Curvature4Act_flg : Outport  Port=2
  VLIC_LaneWidth4Act_flg : Outport  Port=3
  VLIC_Heading4Act_flg : Outport  Port=4
  VLIC_Curvature4Disable_flg : Outport  Port=5
  VLIC_TLCLTrigger_flg : Outport  Port=6
  VLIC_TLCRTrigger_flg : Outport  Port=7
  VLIC_LeftLaneCrossing_flg : Outport  Port=8
  VLIC_RightLaneCrossing_flg : Outport  Port=9
  VLIC_Curvature4DisableWarning_flg : Outport  Port=10
  VLIC_ResidualLaneExhaust_flg : Outport  Port=11
  VLIC_DegradedFinish_flg : Outport  Port=12
  wires:
  KLIC_C1Max4Act_rad/1 -> Relational Operator18/2
  Relational Operator21/1 -> VLIC_Heading4Act_flg/1  "VLIC_Heading4Act_flg"
  "KLIC_Lane4ActThr_sec   "/1 -> Relational Operator21/2
  Timer6/1 -> Relational Operator21/1
  Logical Operator5/1 -> Timer6/Enable
  Relational Operator20/1 -> Logical Operator5/2
  Relational Operator18/1 -> Logical Operator5/1
  "KLIC_C1Max4Act_rad "/1 -> Relational Operator20/2
  VLIC_LaneC1R_rad/1 -> [VLIC_LaneC1R_rad], Abs3/1
  VLIC_LaneC1L_rad/1 -> [VLIC_LaneC1L_rad], Abs2/1
  Add/1 -> IsInRange/1
  Relational Operator19/1 -> VLIC_LaneWidth4Act_flg/1  "VLIC_LaneWidth4Act_flg"
  VLIC_LaneC0R_m/1 -> [VLIC_LaneC0R_m], Add/2
  "KLIC_Lane4ActThr_sec "/1 -> Relational Operator19/2
  Timer5/1 -> Relational Operator19/1
  VLIC_LaneC0L_m/1 -> [VLIC_LaneC0L_m], Add/1
  Relational Operator4/1 -> VLIC_Curvature4Disable_flg/1  "VLIC_Curvature4Disable_flg"
  Logical Operator6/1 -> VLIC_LaneNotAvail_flg/1  "VLIC_LaneNotAvail_flg"
  KLIC_C2Max4DisableThr_sec/1 -> Relational Operator17/2
  Timer4/1 -> Relational Operator17/1
  Logical Operator9/1 -> Timer4/Enable
  Relational Operator16/1 -> Logical Operator9/2
  Relational Operator15/1 -> Logical Operator9/1
  "KLIC_C2Max4Disable_rat "/1 -> Relational Operator16/2
  KLIC_C2Max4Disable_rat/1 -> Relational Operator15/2
  KLIC_C2Max4Act_rat/1 -> Relational Operator12/2
  Relational Operator14/1 -> VLIC_Curvature4Act_flg/1  "VLIC_Curvature4Act_flg"
  KLIC_Lane4ActThr_sec/1 -> Relational Operator14/2
  Timer3/1 -> Relational Operator14/1
  Logical Operator7/1 -> Timer3/Enable
  Relational Operator12/1 -> Logical Operator7/1
  "KLIC_C2Max4Act_rat "/1 -> Relational Operator3/2
  VLIC_LaneC2L_rat/1 -> Gain5/1
  KLIC_LaneWidthUpThr_m/1 -> IsInRange/2
  KLIC_LaneWidthLowThr_m/1 -> IsInRange/3
  IsInRange/1 -> Timer5/Enable
  VLIC_TLCL_s/1 -> Abs1/1
  VLIC_TLCR_s/1 -> Abs4/1
  "VLIC_RightLaneAvail_fig "/1 -> Logical Operator11/1
  "VLIC_LeftLaneAvail_fig "/1 -> Logical Operator10/1
  Logical Operator10/1 -> Logical Operator6/1
  Logical Operator11/1 -> Logical Operator6/2
  [VLIC_LaneC2LABS_rat] -> Relational Operator15/1
  [VLIC_LaneC2RABS_rat] -> Relational Operator16/1
  Abs1/1 -> Hysteresis_LessThan/1
  Lookup2D/1 -> Sum/1, Hysteresis_LessThan/2
  Sum/1 -> Hysteresis_LessThan/3
  KLIC_TLCTriggerThrHysis_s/1 -> Sum/2
  Hysteresis_LessThan/1 -> VLIC_TLCLTrigger_flg/1  "VLIC_TLCLTrigger_flg"
  Lookup2D1/1 -> Hysteresis_LessThan1/2, Sum1/1
  Sum1/1 -> Hysteresis_LessThan1/3
  "KLIC_TLCTriggerThrHysis_s "/1 -> Sum1/2
  Abs4/1 -> Hysteresis_LessThan1/1
  Hysteresis_LessThan1/1 -> VLIC_TLCRTrigger_flg/1  "VLIC_TLCRTrigger_flg"
  Abs2/1 -> Relational Operator18/1
  Abs3/1 -> Relational Operator20/1
  [VLIC_LaneC1L_rad] -> Gain1/1
  [VLIC_LaneC1R_rad] -> Gain/1
  Gain/1 -> rad2deg1/1
  rad2deg/1 -> Lookup2D/2
  rad2deg1/1 -> Lookup2D1/2
  VDINR_VehSpd_kph/1 -> [VDINR_VehSpd_kph], Lookup2D/1
  [VDINR_VehSpd_kph] -> Lookup2D1/1
  Gain1/1 -> rad2deg/1
  Unit Delay/1 -> Unit Delay1/1, Compare To Zero1/1
  Compare To Zero/1 -> Logical Operator/1
  Compare To Zero1/1 -> Logical Operator/2
  Unit Delay1/1 -> Unit Delay2/1, Compare To Zero2/1
  Unit Delay2/1 -> Compare To Zero3/1
  Compare To Zero2/1 -> Logical Operator/3
  Compare To Zero3/1 -> Logical Operator/4
  Logical Operator/1 -> VLIC_LeftLaneCrossing_flg/1  "VLIC_LeftLaneCrossing_flg"
  Unit Delay3/1 -> Compare To Zero5/1, Unit Delay4/1
  Unit Delay4/1 -> Compare To Zero6/1, Unit Delay5/1
  Unit Delay5/1 -> Compare To Zero7/1
  KAPP_VehicleWidth_m/1 -> Gain2/1
  [VLIC_LaneC0L_m] -> Add1/1
  Gain2/1 -> Add1/2
  "KAPP_VehicleWidth_m "/1 -> Gain3/1
  Gain3/1 -> Add2/2
  [VLIC_LaneC0R_m] -> Add2/1
  Add1/1 -> Relational Operator2/1, Unit Delay/1, Compare To Zero/1
  KLIC_LaneCrossingMinC0_m/1 -> Relational Operator2/2
  Add2/1 -> Compare To Zero4/1, Gain4/1, Unit Delay3/1
  KLIC_LaneCrossingMinC0_m1/1 -> Relational Operator1/2
  Gain4/1 -> Relational Operator1/1
  Abs5/1 -> divide/2
  Constant/1 -> divide/1
  Gain5/1 -> Abs5/1
  Constant1/1 -> divide1/1
  VLIC_LaneC2R_rat/1 -> Gain6/1
  Gain6/1 -> Abs7/1
  Abs7/1 -> divide1/2
  divide1/1 -> Relational Operator3/1, [VLIC_LaneC2RABS_rat]  "VLIC_LaneC2RRadius_m"
  Relational Operator3/1 -> Logical Operator7/2
  divide/1 -> [VLIC_LaneC2LABS_rat], Relational Operator12/1  "VLIC_LaneC2RRadius_m"
  KLIC_C2Max4Act_rat1/1 -> divide/3
  KLIC_C2Max4Act_rat2/1 -> divide1/3
  Relational Operator17/1 -> VLIC_Curvature4DisableWarning_flg/1, Timer1/Enable  "VLIC_Curvature4DisableWarning_flg"
  Timer1/1 -> Relational Operator4/1
  KLIC_C2Max4DisableThr_sec1/1 -> Relational Operator4/2
  Relational Operator2/1 -> Logical Operator/5
  Compare To Zero7/1 -> Logical Operator1/4
  Compare To Zero5/1 -> Logical Operator1/2
  Compare To Zero6/1 -> Logical Operator1/3
  Compare To Zero4/1 -> Logical Operator1/1
  Relational Operator1/1 -> Logical Operator1/5
  Logical Operator1/1 -> VLIC_RightLaneCrossing_flg/1  "VLIC_RightLaneCrossing_flg"
  SR-Latch/1 -> Logical Operator8/1
  Constant2/1 -> Relational Operator6/2, Relational Operator/2
  VLIC_ResidualLaneL_s/1 -> Relational Operator/1
  Timer2/1 -> Relational Operator8/1
  Relational Operator9/1 -> Logical Operator13/2
  Relational Operator6/1 -> Logical Operator2/2
  Logical Operator4/1 -> Logical Operator3/1
  Constant3/1 -> Relational Operator5/2
  Logical Operator8/1 -> VLIC_ResidualLaneExhaust_flg/1  "VLIC_ResidualLaneExhaust_flg"
  Constant4/1 -> Relational Operator7/2
  VLIC_ResidualLaneR_s/1 -> Relational Operator6/1
  Constant7/1 -> Relational Operator10/2
  VLFC_LFCState_enum/1 -> Relational Operator7/1, Relational Operator10/1
  SR-Latch1/1 -> VLIC_DegradedFinish_flg/1  "VLIC_DegradedFinish_flg"
  Logical Operator13/1 -> SR-Latch1/2
  Timer7/1 -> Relational Operator9/1
  Relational Operator10/1 -> Logical Operator8/2
  Relational Operator5/1 -> Logical Operator3/2
  Constant6/1 -> Relational Operator9/2
  Constant5/1 -> Relational Operator8/2
  Relational Operator7/1 -> Timer2/Enable
  Relational Operator8/1 -> SR-Latch1/1, Logical Operator12/1, Timer7/Enable
  Logical Operator3/1 -> SR-Latch/2
  Logical Operator12/1 -> Logical Operator13/1
  Relational Operator/1 -> Logical Operator2/1
  Timer/1 -> Relational Operator5/1
  Logical Operator2/1 -> Logical Operator4/1, Timer/Enable, SR-Latch/1

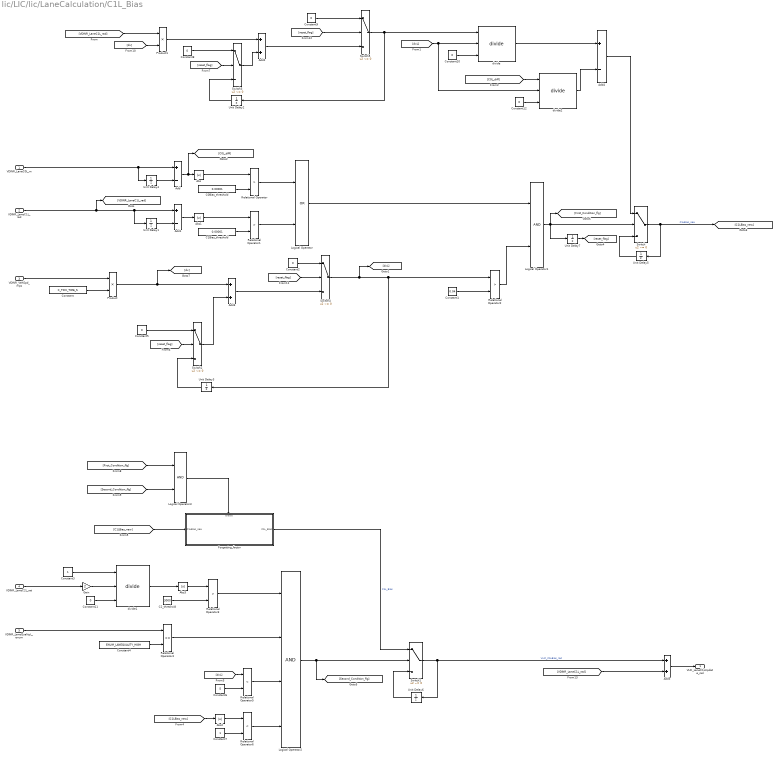
== system lic/LIC/lic/LaneCalculation/C1L_Bias ==
  VDINR_LaneC0L_m : Inport
  VDINR_LaneC1L_rad : Inport  Port=2
  VDINR_VehSpd_mps : Inport  Port=3
  VDINR_LaneC2L_rat : Inport  Port=4
  VDINR_LaneQualityL_enum : Inport  Port=5
  Abs{,1..3} (4 alike) : Abs
  Add : Sum  Inputs=+-
  Add1 : Sum  Inputs=+-
  Add2 : Sum
  Add3 : Sum
  Add4 : Sum  Inputs=+-
  Add5 : Sum
  C0Bias_threshold : Constant  Value=0.00001  OutDataTypeStr=single
  C1Bias_threshold : Constant  Value=0.00001  OutDataTypeStr=single
  C2_threshold : Constant  Value=3000  OutDataTypeStr=single
  Constant : Constant  Value=C_TICK_TIME_S
  Constant1 : Constant  Value=0.04  OutDataTypeStr=single
  Constant{2,5,8..12} (7 alike) : Constant  Value=0  OutDataTypeStr=single
  Constant3 : Constant  OutDataTypeStr=single
  Constant4 : Constant  Value=ENUM_LANEQUALITY_HIGH
  Constant6 : Constant  Value=5  OutDataTypeStr=single
  Constant7 : Constant  OutDataTypeStr=single
  Forgetting_factor : Subsystem  TreatAsAtomicUnit=on
  Gain : Gain  Gain=2
  Logical Operator : Logic  Operator=OR  AllPortsSameDT=off  OutDataTypeStr=boolean
  Logical Operator1 : Logic  AllPortsSameDT=off  OutDataTypeStr=boolean
  Logical Operator2 : Logic  Inputs=4  AllPortsSameDT=off  OutDataTypeStr=boolean
  Logical Operator3 : Logic  AllPortsSameDT=off  OutDataTypeStr=boolean
  Product : Product
  Product1 : Product
  Relational Operator{,1..3} (4 alike) : RelationalOperator  Operator=>  OutDataTypeStr=boolean  RndMeth=Nearest
  Relational Operator4 : RelationalOperator  Operator===  OutDataTypeStr=boolean  RndMeth=Nearest
  Relational Operator5 : RelationalOperator  Operator=<  OutDataTypeStr=boolean  RndMeth=Nearest
  Relational Operator6 : RelationalOperator  Operator=<  OutDataTypeStr=boolean  RndMeth=Nearest
  Switch{,1..5} (6 alike) : Switch  Criteria=u2 ~= 0
  Unit Delay{1..7} (7 alike) : UnitDelay  SampleTime=-1  HasFrameUpgradeWarning=on
  divide : hcu_lib/divide
  divide1 : hcu_lib/divide
  divide2 : hcu_lib/divide
  VLIC_LaneC1LUpdate_rad : Outport
  wires:
  Add5/1 -> VLIC_LaneC1LUpdate_rad/1
  [VDINR_LaneC1L_rad] -> Add5/2
  VDINR_LaneC0L_m/1 -> Unit Delay4/1, Add/1
  Unit Delay4/1 -> Add/2
  VDINR_LaneC1L_rad/1 -> [VDINR_LaneC1L_rad], Unit Delay1/1, Add1/1
  Unit Delay1/1 -> Add1/2
  Add/1 -> [C0L_diff], Abs/1
  Add1/1 -> Abs1/1
  VDINR_VehSpd_mps/1 -> Product/1
  Abs/1 -> Relational Operator/1
  C0Bias_threshold/1 -> Relational Operator/2
  Abs1/1 -> Relational Operator1/1
  C1Bias_threshold/1 -> Relational Operator1/2
  Add3/1 -> Switch4/3
  Constant1/1 -> Relational Operator2/2
  Relational Operator/1 -> Logical Operator/1
  Relational Operator1/1 -> Logical Operator/2
  Logical Operator/1 -> Logical Operator1/1
  Relational Operator2/1 -> Logical Operator1/2
  Logical Operator1/1 -> Switch/2, [First_Condition_flg], Unit Delay7/1
  [dx] -> Product1/2
  [VDINR_LaneC1L_rad] -> Product1/1
  Product1/1 -> Add2/1
  Constant/1 -> Product/2
  Product/1 -> [dx], Add3/1
  [dxL] -> divide2/2, divide/2
  divide/1 -> Add4/1
  [C0L_diff] -> divide2/1
  divide2/1 -> Add4/2
  Add4/1 -> Switch/1
  VDINR_LaneC2L_rat/1 -> Gain/1
  C2_threshold/1 -> Relational Operator3/2
  VDINR_LaneQualityL_enum/1 -> Relational Operator4/1
  Constant4/1 -> Relational Operator4/2
  Relational Operator3/1 -> Logical Operator2/1
  Relational Operator4/1 -> Logical Operator2/2
  [dxL] -> Relational Operator5/1
  Constant6/1 -> Relational Operator5/2
  Relational Operator5/1 -> Logical Operator2/3
  Relational Operator6/1 -> Logical Operator2/4
  Switch/1 -> Unit Delay5/1, [C1LBias_new]  "C1LBias_new"
  Switch1/1 -> Add5/1, Unit Delay6/1  "VLIC_C1LBias_rad"
  [C1LBias_new] -> Abs2/1
  Abs2/1 -> Relational Operator6/1
  Constant7/1 -> Relational Operator6/2
  Forgetting_factor/1(C1L_Bias) -> Switch1/1  "C1L_Bias"
  [C1LBias_new] -> Forgetting_factor/1(C1LBias_new)
  Unit Delay5/1 -> Switch/3
  Unit Delay6/1 -> Switch1/3
  Abs3/1 -> Relational Operator3/1
  Logical Operator2/1 -> [Second_Condition_flg], Switch1/2
  Switch2/1 -> Add3/2
  Constant5/1 -> Switch2/1
  [reset_flag] -> Switch2/2
  Constant8/1 -> Switch3/1
  [reset_flag] -> Switch3/2
  Switch3/1 -> Add2/2
  Unit Delay7/1 -> [reset_flag]
  Unit Delay2/1 -> Switch3/3
  Unit Delay3/1 -> Switch2/3
  [First_Condition_flg] -> Logical Operator3/1
  [Second_Condition_flg] -> Logical Operator3/2
  Logical Operator3/1 -> Forgetting_factor/Enable
  [reset_flag] -> Switch4/2
  Constant2/1 -> Switch4/1
  Switch4/1 -> [dxL], Unit Delay3/1, Relational Operator2/1
  Add2/1 -> Switch5/3
  [reset_flag] -> Switch5/2
  Constant9/1 -> Switch5/1
  Switch5/1 -> divide/1, Unit Delay2/1
  Constant10/1 -> divide/3
  divide1/1 -> Abs3/1
  Constant3/1 -> divide1/1
  Gain/1 -> divide1/2
  Constant11/1 -> divide1/3
  Constant12/1 -> divide2/3

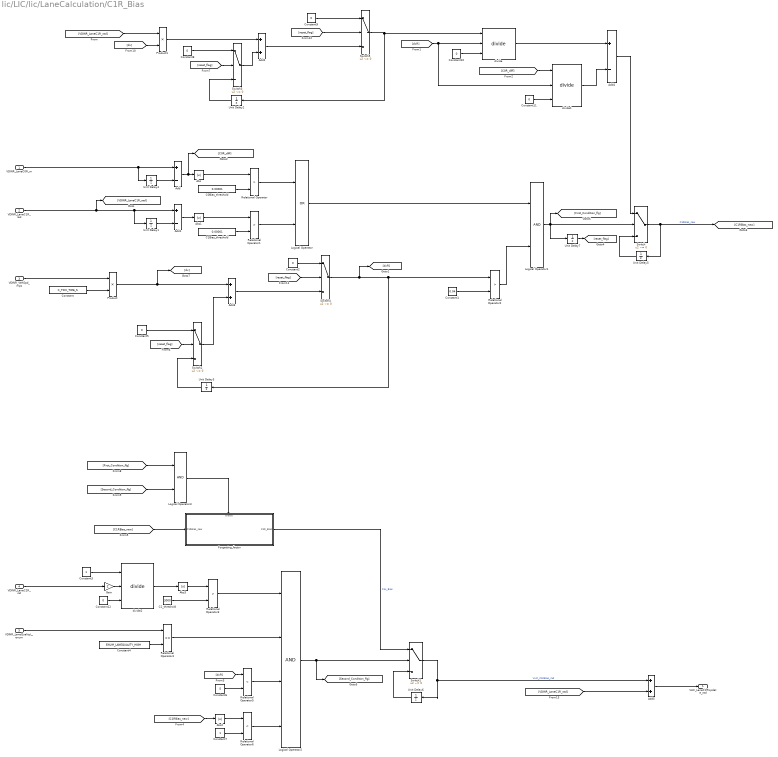
== system lic/LIC/lic/LaneCalculation/C1R_Bias ==
  VDINR_LaneC0R_m : Inport
  VDINR_LaneC1R_rad : Inport  Port=2
  VDINR_VehSpd_mps : Inport  Port=3
  VDINR_LaneC2R_rat : Inport  Port=4
  VDINR_LaneQualityL_enum : Inport  Port=5
  Abs{,1..3} (4 alike) : Abs
  Add : Sum  Inputs=+-
  Add1 : Sum  Inputs=+-
  Add2 : Sum
  Add3 : Sum
  Add4 : Sum  Inputs=+-
  Add5 : Sum
  C0Bias_threshold : Constant  Value=0.00001  OutDataTypeStr=single
  C1Bias_threshold : Constant  Value=0.00001  OutDataTypeStr=single
  C2_threshold : Constant  Value=3000  OutDataTypeStr=single
  Constant : Constant  Value=C_TICK_TIME_S
  Constant1 : Constant  Value=0.04  OutDataTypeStr=single
  Constant{2,5,8..12} (7 alike) : Constant  Value=0  OutDataTypeStr=single
  Constant3 : Constant  OutDataTypeStr=single
  Constant4 : Constant  Value=ENUM_LANEQUALITY_HIGH
  Constant6 : Constant  Value=5  OutDataTypeStr=single
  Constant7 : Constant  OutDataTypeStr=single
  Forgetting_factor : Subsystem  TreatAsAtomicUnit=on
  Gain : Gain  Gain=2
  Logical Operator : Logic  Operator=OR  AllPortsSameDT=off  OutDataTypeStr=boolean
  Logical Operator1 : Logic  AllPortsSameDT=off  OutDataTypeStr=boolean
  Logical Operator2 : Logic  Inputs=4  AllPortsSameDT=off  OutDataTypeStr=boolean
  Logical Operator3 : Logic  AllPortsSameDT=off  OutDataTypeStr=boolean
  Product : Product
  Product1 : Product
  Relational Operator{,1..3} (4 alike) : RelationalOperator  Operator=>  OutDataTypeStr=boolean  RndMeth=Nearest
  Relational Operator4 : RelationalOperator  Operator===  OutDataTypeStr=boolean  RndMeth=Nearest
  Relational Operator5 : RelationalOperator  Operator=<  OutDataTypeStr=boolean  RndMeth=Nearest
  Relational Operator6 : RelationalOperator  Operator=<  OutDataTypeStr=boolean  RndMeth=Nearest
  Switch{,1..5} (6 alike) : Switch  Criteria=u2 ~= 0
  Unit Delay{1..7} (7 alike) : UnitDelay  SampleTime=-1  HasFrameUpgradeWarning=on
  divide : hcu_lib/divide
  divide1 : hcu_lib/divide
  divide2 : hcu_lib/divide
  VLIC_LaneC1RUpdate_rad : Outport
  wires:
  Add5/1 -> VLIC_LaneC1RUpdate_rad/1
  [VDINR_LaneC1R_rad] -> Add5/2
  VDINR_LaneC0R_m/1 -> Unit Delay4/1, Add/1
  Unit Delay4/1 -> Add/2
  VDINR_LaneC1R_rad/1 -> [VDINR_LaneC1R_rad], Unit Delay1/1, Add1/1
  Unit Delay1/1 -> Add1/2
  Add/1 -> [C0R_diff], Abs/1
  Add1/1 -> Abs1/1
  VDINR_VehSpd_mps/1 -> Product/1
  Abs/1 -> Relational Operator/1
  C0Bias_threshold/1 -> Relational Operator/2
  Abs1/1 -> Relational Operator1/1
  C1Bias_threshold/1 -> Relational Operator1/2
  Add3/1 -> Switch4/3
  Constant1/1 -> Relational Operator2/2
  Relational Operator/1 -> Logical Operator/1
  Relational Operator1/1 -> Logical Operator/2
  Logical Operator/1 -> Logical Operator1/1
  Relational Operator2/1 -> Logical Operator1/2
  Logical Operator1/1 -> Switch/2, [First_Condition_flg], Unit Delay7/1
  [dx] -> Product1/2
  [VDINR_LaneC1R_rad] -> Product1/1
  Product1/1 -> Add2/1
  Constant/1 -> Product/2
  Product/1 -> [dx], Add3/1
  [dxR] -> divide1/2, divide/2
  divide/1 -> Add4/1
  [C0R_diff] -> divide1/1
  divide1/1 -> Add4/2
  Add4/1 -> Switch/1
  VDINR_LaneC2R_rat/1 -> Gain/1
  divide2/1 -> Abs3/1
  C2_threshold/1 -> Relational Operator3/2
  VDINR_LaneQualityL_enum/1 -> Relational Operator4/1
  Constant4/1 -> Relational Operator4/2
  Relational Operator3/1 -> Logical Operator2/1
  Relational Operator4/1 -> Logical Operator2/2
  [dxR] -> Relational Operator5/1
  Constant6/1 -> Relational Operator5/2
  Relational Operator5/1 -> Logical Operator2/3
  Relational Operator6/1 -> Logical Operator2/4
  Switch/1 -> Unit Delay5/1, [C1RBias_new]  "C1RBias_new"
  Switch1/1 -> Unit Delay6/1, Add5/1  "VLIC_C1RBias_rad"
  [C1RBias_new] -> Abs2/1
  Abs2/1 -> Relational Operator6/1
  Constant7/1 -> Relational Operator6/2
  Forgetting_factor/1(C1R_Bias) -> Switch1/1  "C1L_Bias"
  [C1RBias_new] -> Forgetting_factor/1(C1RBias_new)
  Unit Delay5/1 -> Switch/3
  Unit Delay6/1 -> Switch1/3
  Abs3/1 -> Relational Operator3/1
  Logical Operator2/1 -> [Second_Condition_flg], Switch1/2
  Switch2/1 -> Add3/2
  Constant5/1 -> Switch2/1
  [reset_flag] -> Switch2/2
  Constant8/1 -> Switch3/1
  [reset_flag] -> Switch3/2
  Switch3/1 -> Add2/2
  Unit Delay7/1 -> [reset_flag]
  Unit Delay2/1 -> Switch3/3
  Unit Delay3/1 -> Switch2/3
  [First_Condition_flg] -> Logical Operator3/1
  [Second_Condition_flg] -> Logical Operator3/2
  Logical Operator3/1 -> Forgetting_factor/Enable
  [reset_flag] -> Switch4/2
  Constant2/1 -> Switch4/1
  Switch4/1 -> [dxR], Unit Delay3/1, Relational Operator2/1
  Add2/1 -> Switch5/3
  [reset_flag] -> Switch5/2
  Constant9/1 -> Switch5/1
  Switch5/1 -> divide/1, Unit Delay2/1
  Constant10/1 -> divide/3
  Constant11/1 -> divide1/3
  Constant3/1 -> divide2/1
  Gain/1 -> divide2/2
  Constant12/1 -> divide2/3

== system lic/LIC/lic/LaneCalculation/GenerateLeftLane ==
  VDINR_LaneC0L_m : Inport
  VLIC_EstLaneC0L_m : Inport  Port=2
  VDINR_LaneC1L_rad : Inport  Port=3
  VLIC_EstLaneC1L_rad : Inport  Port=4
  VDINR_LaneC2L_rat : Inport  Port=5
  VLIC_EstLaneC2L_rat : Inport  Port=6
  VDINR_LaneC3L_rat : Inport  Port=7
  VLIC_EstLaneC3L_rat : Inport  Port=8
  VLIC_LeftLaneAvail_flg : Inport  Port=9
  Switch{3,12..14} (4 alike) : Switch  Criteria=u2 ~= 0
  VLIC_LaneC0L_m : Outport
  VLIC_LaneC1L_rad : Outport  Port=2
  VLIC_LaneC2L_rat : Outport  Port=3
  VLIC_LaneC3L_rat : Outport  Port=4
  wires:
  VLIC_EstLaneC0L_m/1 -> Switch3/3
  Switch12/1 -> VLIC_LaneC1L_rad/1  "VLIC_LaneC1L_rad"
  VLIC_EstLaneC1L_rad/1 -> Switch12/3
  VDINR_LaneC1L_rad/1 -> Switch12/1
  Switch3/1 -> VLIC_LaneC0L_m/1  "VLIC_LaneC0L_m"
  Switch13/1 -> VLIC_LaneC2L_rat/1  "VLIC_LaneC2L_rat"
  VLIC_EstLaneC2L_rat/1 -> Switch13/3
  VDINR_LaneC2L_rat/1 -> Switch13/1
  VLIC_LeftLaneAvail_flg/1 -> Switch14/2, Switch13/2, Switch12/2, Switch3/2
  VLIC_EstLaneC3L_rat/1 -> Switch14/3
  VDINR_LaneC3L_rat/1 -> Switch14/1
  VDINR_LaneC0L_m/1 -> Switch3/1
  Switch14/1 -> VLIC_LaneC3L_rat/1  "VLIC_LaneC3L_rat"
